simulink model "Project"  (R2016a)
settings: Solver=VariableStepAuto  StartTime=0.0  StopTime=10.0  RelTol=1e-3
libraries: dsparch4 x2
settings Model: Creator=DELL  LastModifiedBy=DELL

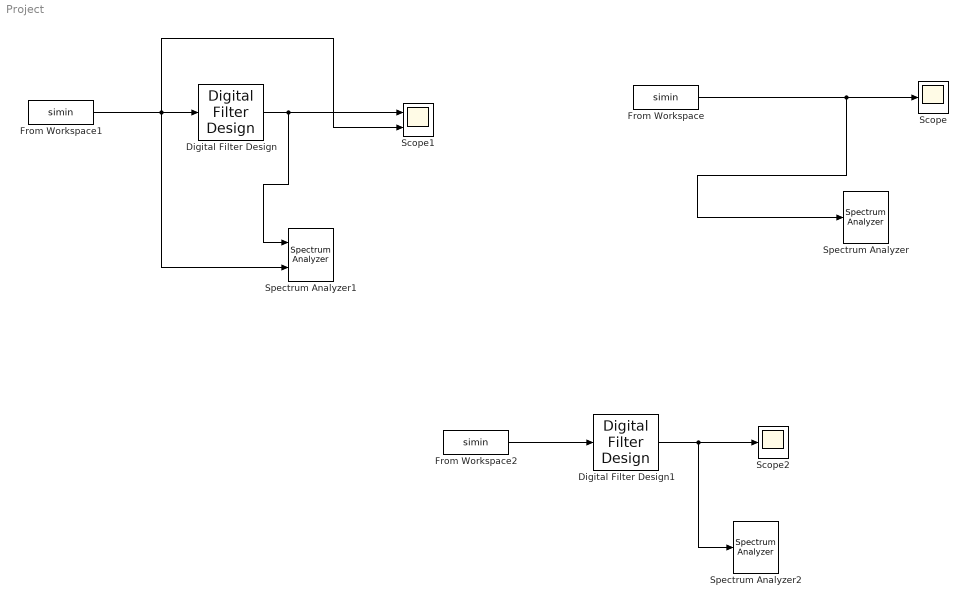
== system Project ==
  Digital Filter Design : dsparch4/Digital Filter Design  mwdsp_browser_bugfix_var=off
  Digital Filter Design1 : dsparch4/Digital Filter Design  mwdsp_browser_bugfix_var=off
  From Workspace : FromWorkspace  VariableName=simin  SampleTime=1/256
  From Workspace1 : FromWorkspace  VariableName=simin  SampleTime=1/256
  From Workspace2 : FromWorkspace  VariableName=simin  SampleTime=1/256
  Scope : Scope
  Scope1 : Scope  NumInputPorts=2
  Scope2 : Scope
  Spectrum Analyzer : SpectrumAnalyzer
  Spectrum Analyzer1 : SpectrumAnalyzer  NumInputPorts=2
  Spectrum Analyzer2 : SpectrumAnalyzer
  wires:
  From Workspace/1 -> Spectrum Analyzer/1, Scope/1
  From Workspace1/1 -> Scope1/2, Spectrum Analyzer1/2, Digital Filter Design/1
  Digital Filter Design/1 -> Spectrum Analyzer1/1, Scope1/1
  From Workspace2/1 -> Digital Filter Design1/1
  Digital Filter Design1/1 -> Spectrum Analyzer2/1, Scope2/1
